simulink model "vkrzam"  (R2023b)
settings: Solver=ode5  StartTime=0.0  StopTime=2000  FixedStep=0.1  RelTol=1e-3
libraries: slpidlib x2
settings Model: Creator=Анастасия  LastModifiedBy=Анастасия

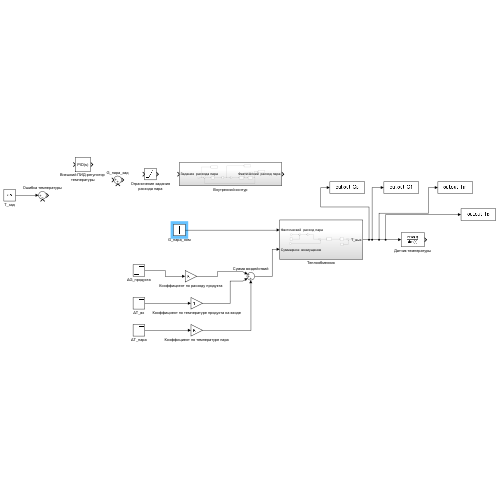
[thumbnail: Simulink's stored preview of the top-level diagram]
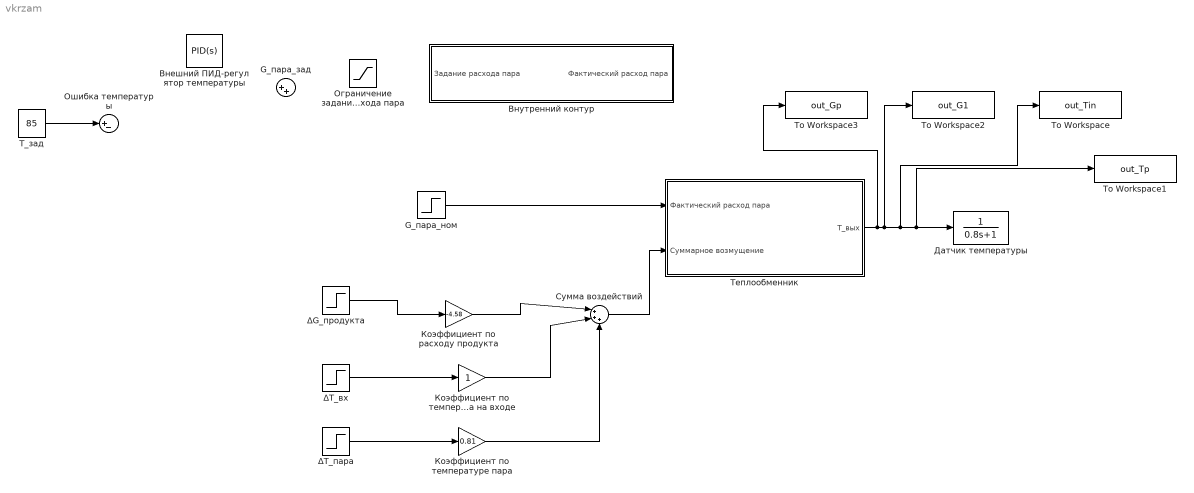
== system vkrzam ==
  G_пара_зад : Sum  Inputs=|++
  G_пара_ном : Step  Time=300  Before=0.67  After=0.67  SampleTime=0
  T_зад : Constant  Value=85
  To Workspace : ToWorkspace  VariableName=out_Tin  SaveFormat=Timeseries  SampleTime=0.5
  To Workspace1 : ToWorkspace  VariableName=out_Tp  SaveFormat=Timeseries  SampleTime=0.5
  To Workspace2 : ToWorkspace  VariableName=out_G1  SaveFormat=Timeseries  SampleTime=0.5
  To Workspace3 : ToWorkspace  VariableName=out_Gp  SaveFormat=Timeseries  SampleTime=0.5
  ΔG_продукта : Step  Time=300  After=0  SampleTime=0
  ΔT_вх : Step  Time=300  After=0  SampleTime=0
  ΔT_пара : Step  Time=300  After=4.0  SampleTime=0
  Внешний ПИД-регулятор температуры : slpidlib/PID Controller  Controller=PID  Form=Parallel  TimeDomain=Continuous-time  UseExternalTs=off  SampleTime=-1  IntegratorMethod=Forward Euler  FilterMethod=Forward Euler  ControllerParametersSource=internal  P=0.016  I=0.0004  UseKiTs=off  D=0.1  N=10  UseFilter=on  TunerSelectOption=Transfer Function Based (PID Tuner App)  InitialConditionSource=internal  InitialConditionForIntegrator=0  InitialConditionForFilter=0  DifferentiatorICPrevScaledInput=0  ExternalReset=none  TrackingMode=off  Kt=1  LimitOutput=off  SatLimitsSource=internal  UpperSaturationLimit=inf  LowerSaturationLimit=-inf  LinearizeAsGain=on  AntiWindupMode=none  Kb=1  LimitIntegrator=off  UpperIntegratorSaturationLimit=inf  LowerIntegratorSaturationLimit=-inf  POutMin=[]  POutMax=[]  IOutMin=[]  IOutMax=[]  DOutMin=[]  DOutMax=[]  NOutMin=[]  NOutMax=[]  SumOutMin=[]  SumOutMax=[]  SaturationOutMin=[]  SaturationOutMax=[]  PParamMin=[]  PParamMax=[]  IParamMin=[]  IParamMax=[]  DParamMin=[]  DParamMax=[]  NParamMin=[]  NParamMax=[]  KbParamMin=[]  KbParamMax=[]  KtParamMin=[]  KtParamMax=[]  KbOutMin=[]  KbOutMax=[]  KtOutMin=[]  KtOutMax=[]  IntegratorOutMin=[]  IntegratorOutMax=[]  FilterOutMin=[]  FilterOutMax=[]  SumI1OutMin=[]  SumI1OutMax=[]  SumI2OutMin=[]  SumI2OutMax=[]  SumI3OutMin=[]  SumI3OutMax=[]  SumI4OutMin=[]  SumI4OutMax=[]  SumDOutMin=[]  SumDOutMax=[]  DifferentiatorOutMin=[]  DifferentiatorOutMax=[]  FilterDiffOutCoefMin=[]  FilterDiffOutCoefMax=[]  ReciprocalOutMin=[]  ReciprocalOutMax=[]  SumDenOutMin=[]  SumDenOutMax=[]  SumNumOutMin=[]  SumNumOutMax=[]  DivideOutMin=[]  DivideOutMax=[]  UdiffTsProdOutMin=[]  UdiffTsProdOutMax=[]  NTsProdOutMin=[]  NTsProdOutMax=[]  UintegralTsProdOutMin=[]  UintegralTsProdOutMax=[]  UngainTsProdOutMin=[]  UngainTsProdOutMax=[]  ClampingZeroOutDataTypeStr=Inherit: Inherit via back propagation  ClampingZeroOutMin=[]  ClampingZeroOutMax=[]  FilterDenConstantOutDataTypeStr=Inherit: Inherit via back propagation  FilterDenConstantOutMin=[]  FilterDenConstantOutMax=[]  PCopyOutDataTypeStr=Inherit: Inherit via back propagation  PCopyOutMin=[]  PCopyOutMax=[]  NCopyOutDataTypeStr=Inherit: Inherit via back propagation  NCopyOutMin=[]  NCopyOutMax=[]  IntegratorContinuousStateAttributes=''  IntegratorStateMustResolveToSignalObject=off  IntegratorRTWStateStorageClass=Auto  FilterContinuousStateAttributes=''  FilterStateMustResolveToSignalObject=off  FilterRTWStateStorageClass=Auto  ParallelPVariant=InternalParameters  IdealPVariant=Disabled  IVariant=InternalParameters  DVariant=InternalParameters  IntegratorVariant=Continuous  SatVariant=Disabled  AWVariant=Passthrough  PCopyVariant=Disabled  TRVariant=Disabled  FdbkBlocksVariant=Forward  IdealPFdbkVariant=Disabled  SatFdbkVariant=Disabled  DerivativeFilterVariant=ContFilter  NVariant=InternalParameters  NCopyVariant=Disabled  FilterICVariant=InternalICsFilter  IntegratorICVariant=InternalICs  ExternalResetVariant=Disabled  TRSumVariant=Passthrough  SumFdbkVariant=Disabled  SumVariant=Sum_PID  TsampFilterVariant=InternalTs  TsampNgainVariant=Passthrough  TsampIntegralVariant=Disabled_SignalSpec  ExternalSaturationOutDataTypeStr=Inherit: Same as second input
  Внутренний контур : Subsystem
  Датчик температуры : TransferFcn  Denominator=[0.8 1]
  Коэффициент по расходу продукта : Gain  Gain=-4.58
  Коэффициент по температуре пара : Gain  Gain=0.81
  Коэффициент по температуре продукта на входе : Gain
  Ограничение задания расхода пара : Saturate  UpperLimit=1.5  LowerLimit=0
  Ошибка температуры : Sum  Inputs=|+-
  Сумма воздействий : Sum  Inputs=|+++
  Теплообменник : Subsystem
  wires:
  Коэффициент по температуре пара/1 -> Сумма воздействий/3
  T_зад/1 -> Ошибка температуры/1
  ΔT_пара/1 -> Коэффициент по температуре пара/1
  Теплообменник/1(T_вых) -> To Workspace3/1, To Workspace2/1, To Workspace/1, To Workspace1/1, Датчик температуры/1
  Коэффициент по расходу продукта/1 -> Сумма воздействий/1
  Коэффициент по температуре продукта на входе/1 -> Сумма воздействий/2
  ΔT_вх/1 -> Коэффициент по температуре продукта на входе/1
  ΔG_продукта/1 -> Коэффициент по расходу продукта/1
  Сумма воздействий/1 -> Теплообменник/2(Cуммарное возмущение)
  G_пара_ном/1 -> Теплообменник/1(Фактический расход пара)

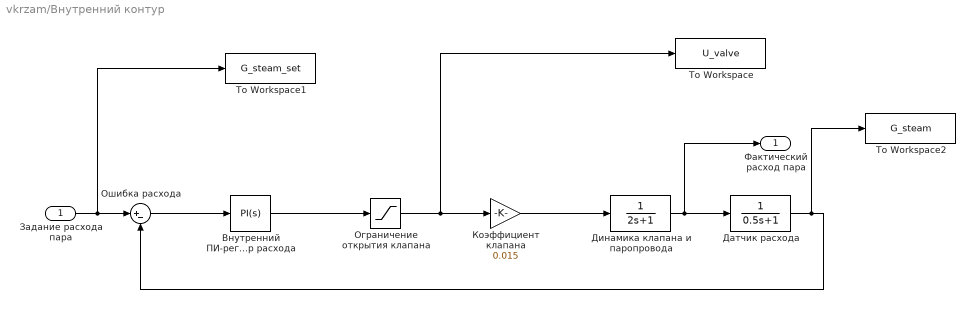
== system vkrzam/Внутренний контур ==
  Задание расхода пара : Inport
  To Workspace : ToWorkspace  VariableName=U_valve  SaveFormat=Timeseries  SampleTime=-1
  To Workspace1 : ToWorkspace  VariableName=G_steam_set  SaveFormat=Timeseries  SampleTime=-1
  To Workspace2 : ToWorkspace  VariableName=G_steam  SaveFormat=Timeseries  SampleTime=-1
  Внутренний ПИ-регулятор расхода : slpidlib/PID Controller  Controller=PI  Form=Parallel  TimeDomain=Continuous-time  UseExternalTs=off  SampleTime=-1  IntegratorMethod=Forward Euler  FilterMethod=Forward Euler  ControllerParametersSource=internal  P=40  I=30  UseKiTs=off  D=0  N=100  UseFilter=on  TunerSelectOption=Transfer Function Based (PID Tuner App)  InitialConditionSource=internal  InitialConditionForIntegrator=0  InitialConditionForFilter=0  DifferentiatorICPrevScaledInput=0  ExternalReset=none  TrackingMode=off  Kt=1  LimitOutput=off  SatLimitsSource=internal  UpperSaturationLimit=inf  LowerSaturationLimit=-inf  LinearizeAsGain=on  AntiWindupMode=none  Kb=1  LimitIntegrator=off  UpperIntegratorSaturationLimit=inf  LowerIntegratorSaturationLimit=-inf  POutMin=[]  POutMax=[]  IOutMin=[]  IOutMax=[]  DOutMin=[]  DOutMax=[]  NOutMin=[]  NOutMax=[]  SumOutMin=[]  SumOutMax=[]  SaturationOutMin=[]  SaturationOutMax=[]  PParamMin=[]  PParamMax=[]  IParamMin=[]  IParamMax=[]  DParamMin=[]  DParamMax=[]  NParamMin=[]  NParamMax=[]  KbParamMin=[]  KbParamMax=[]  KtParamMin=[]  KtParamMax=[]  KbOutMin=[]  KbOutMax=[]  KtOutMin=[]  KtOutMax=[]  IntegratorOutMin=[]  IntegratorOutMax=[]  FilterOutMin=[]  FilterOutMax=[]  SumI1OutMin=[]  SumI1OutMax=[]  SumI2OutMin=[]  SumI2OutMax=[]  SumI3OutMin=[]  SumI3OutMax=[]  SumI4OutMin=[]  SumI4OutMax=[]  SumDOutMin=[]  SumDOutMax=[]  DifferentiatorOutMin=[]  DifferentiatorOutMax=[]  FilterDiffOutCoefMin=[]  FilterDiffOutCoefMax=[]  ReciprocalOutMin=[]  ReciprocalOutMax=[]  SumDenOutMin=[]  SumDenOutMax=[]  SumNumOutMin=[]  SumNumOutMax=[]  DivideOutMin=[]  DivideOutMax=[]  UdiffTsProdOutMin=[]  UdiffTsProdOutMax=[]  NTsProdOutMin=[]  NTsProdOutMax=[]  UintegralTsProdOutMin=[]  UintegralTsProdOutMax=[]  UngainTsProdOutMin=[]  UngainTsProdOutMax=[]  ClampingZeroOutDataTypeStr=Inherit: Inherit via back propagation  ClampingZeroOutMin=[]  ClampingZeroOutMax=[]  FilterDenConstantOutDataTypeStr=Inherit: Inherit via back propagation  FilterDenConstantOutMin=[]  FilterDenConstantOutMax=[]  PCopyOutDataTypeStr=Inherit: Inherit via back propagation  PCopyOutMin=[]  PCopyOutMax=[]  NCopyOutDataTypeStr=Inherit: Inherit via back propagation  NCopyOutMin=[]  NCopyOutMax=[]  IntegratorContinuousStateAttributes=''  IntegratorStateMustResolveToSignalObject=off  IntegratorRTWStateStorageClass=Auto  FilterContinuousStateAttributes=''  FilterStateMustResolveToSignalObject=off  FilterRTWStateStorageClass=Auto  ParallelPVariant=InternalParameters  IdealPVariant=Disabled  IVariant=InternalParameters  DVariant=Disabled  IntegratorVariant=Continuous  SatVariant=Disabled  AWVariant=Passthrough  PCopyVariant=Disabled  TRVariant=Disabled  FdbkBlocksVariant=Forward  IdealPFdbkVariant=Disabled  SatFdbkVariant=Disabled  DerivativeFilterVariant=Disabled  NVariant=Disabled  NCopyVariant=Disabled_SignalSpec  FilterICVariant=Disabled  IntegratorICVariant=InternalICs  ExternalResetVariant=Disabled  TRSumVariant=Passthrough  SumFdbkVariant=Disabled  SumVariant=Sum_PI  TsampFilterVariant=InternalTs  TsampNgainVariant=Passthrough  TsampIntegralVariant=Disabled_SignalSpec  ExternalSaturationOutDataTypeStr=Inherit: Same as second input
  Датчик расхода : TransferFcn  Denominator=[0.5,1]
  Динамика клапана и паропровода : TransferFcn  Denominator=[2 1]
  Коэффициент клапана : Gain  Gain=0.015
  Ограничение открытия клапана : Saturate  UpperLimit=100  LowerLimit=0
  Ошибка расхода : Sum  Inputs=|+-
  Фактический расход пара : Outport
  wires:
  Динамика клапана и паропровода/1 -> Фактический расход пара/1, Датчик расхода/1
  Коэффициент клапана/1 -> Динамика клапана и паропровода/1
  Ошибка расхода/1 -> Внутренний ПИ-регулятор расхода/1
  Внутренний ПИ-регулятор расхода/1 -> Ограничение открытия клапана/1
  Задание расхода пара/1 -> To Workspace1/1, Ошибка расхода/1
  Датчик расхода/1 -> To Workspace2/1, Ошибка расхода/2
  Ограничение открытия клапана/1 -> To Workspace/1, Коэффициент клапана/1

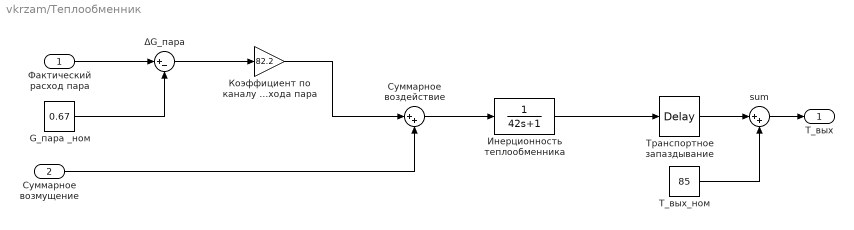
== system vkrzam/Теплообменник ==
  Фактический расход пара : Inport
  Cуммарное возмущение : Inport  Port=2
  "  sum" : Sum  Inputs=|++
  G_пара _ном : Constant  Value=0.67
  T_вых_ном : Constant  Value=85
  ΔG_пара : Sum  Inputs=|+-
  Инерционность теплообменника : TransferFcn  Denominator=[42 1]
  Коэффициент по каналу расхода пара : Gain  Gain=82.2
  Суммарное воздействие : Sum  Inputs=|++
  Транспортное запаздывание : TransportDelay  DelayTime=10
  T_вых : Outport
  wires:
  Фактический расход пара/1 -> ΔG_пара/1
  G_пара _ном/1 -> ΔG_пара/2
  ΔG_пара/1 -> Коэффициент по каналу расхода пара/1
  Cуммарное возмущение/1 -> Суммарное воздействие/2
  Коэффициент по каналу расхода пара/1 -> Суммарное воздействие/1
  Суммарное воздействие/1 -> Инерционность теплообменника/1
  Инерционность теплообменника/1 -> Транспортное запаздывание/1
  Транспортное запаздывание/1 -> "  sum"/1
  T_вых_ном/1 -> "  sum"/2
  "  sum"/1 -> T_вых/1
